simulink model "kuramoto"  (Simulink 7.4)
settings: Solver=ode45  StartTime=0.0  StopTime=10.0  RelTol=1e-3
undefined symbols (not defined in the file): K, N, omega, rho0, threshold, var
Description:
  | Kuramoto oscillator model
  | copy Jose Rivera
  | chepeadan@gmail.com
settings Model: Creator=chepeadan  LastModifiedBy=chepeadan

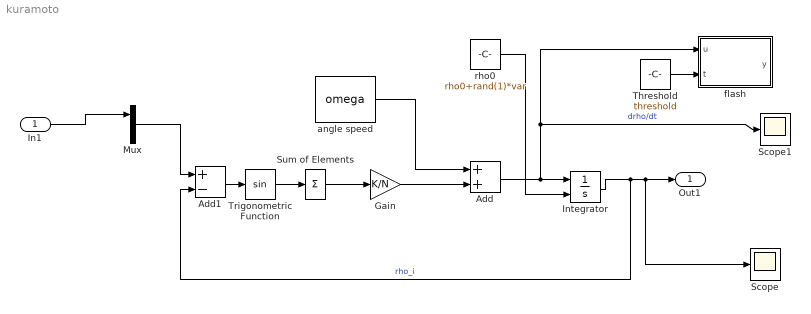
== system kuramoto ==
  In1 : Inport  OutDataType=fixdt(1, 16)  OutScaling=2^0
  Add : Sum  OutDataType=fixdt(1, 16)  OutScaling=2^-10
  Add1 : Sum  Inputs=+-  OutDataType=fixdt(1, 16)  OutScaling=2^-10
  Gain : Gain  Gain=K/N  ParameterDataType=fixdt(1, 16)  ParameterScaling=2^0  OutDataType=fixdt(1, 16)  OutScaling=2^0
  Integrator : Integrator  InitialConditionSource=external
  Mux : Mux  Inputs=2
  Scope : Scope
  Scope1 : Scope
  Sum of Elements : Sum  Inputs=+  OutDataType=fixdt(1, 16)  OutScaling=2^-10
  Threshold : Constant  Value=threshold  OutDataType=fixdt(1, 16)  OutScaling=2^0
  Trigonometric Function : Trigonometry
  angle speed : Constant  Value=omega  OutDataType=fixdt(1, 16)  OutScaling=2^0
  flash : Stateflow chart
  rho0 : Constant  Value=rho0+rand(1)*var  OutDataType=fixdt(1, 16)  OutScaling=2^0
  Out1 : Outport  OutDataType=fixdt(1, 16)  OutScaling=2^0
  wires:
  In1/1 -> Mux/1
  Mux/1 -> Add1/1
  Integrator/1 -> Add1/2, Out1/1, Scope/1  "rho_i"
  Add1/1 -> Trigonometric Function/1
  angle speed/1 -> Add/1
  Gain/1 -> Add/2
  Add/1 -> Integrator/1, flash/1(u), Scope1/1  "drho/dt"
  Trigonometric Function/1 -> Sum of Elements/1
  Sum of Elements/1 -> Gain/1
  Threshold/1 -> flash/2(t)
  rho0/1 -> Integrator/2

== matlab function flash ==
  data: u input double; y output double; t input double
function y = fcn(u,t)
%#eml
% Allows the flashing of the subsystem block after some threshold
eml.extrinsic('set_param','get_param','gcs');

y = u;

if u > t
set_param(get_param(gcs,'parent'),'BackgroundColor','[0.3, 0.9, 0.5]');
else
set_param(get_param(gcs,'parent'),'BackgroundColor','white');
end

y = u;
